simulink model "rigidBodyControl"  (R2016b)
settings: Solver=VariableStepAuto  StartTime=0.0  StopTime=0.4  FixedStep=2e-4  RelTol=1e-3
values from neighbouring files (symbols this model uses):
  denominator = denominator{1}    [mainFeedbackTuning.m]    (also in rigidBodyInit.m)
  denQ = [1 2*wq*0.707 wq*wq]    [rigidBodyInit.m]
  fs = 10000    [mainFeedbackTuning.m]    (also in rigidBodyInit.m = 5000)
  numerator = numerator{1}    [mainFeedbackTuning.m]    (also in rigidBodyInit.m)
  numQ = wq*wq    (= 1421223033.76)    [rigidBodyInit.m]
  Ts = 1/fs    (= 0.0001)    [mainFeedbackTuning.m]    (also in rigidBodyInit.m = 0.0002)
undefined symbols (not defined in the file): m0
libraries: simulink x3, model_controller x1
settings Model: Creator=Dai Luyao  LastModifiedBy=Dai Luyao

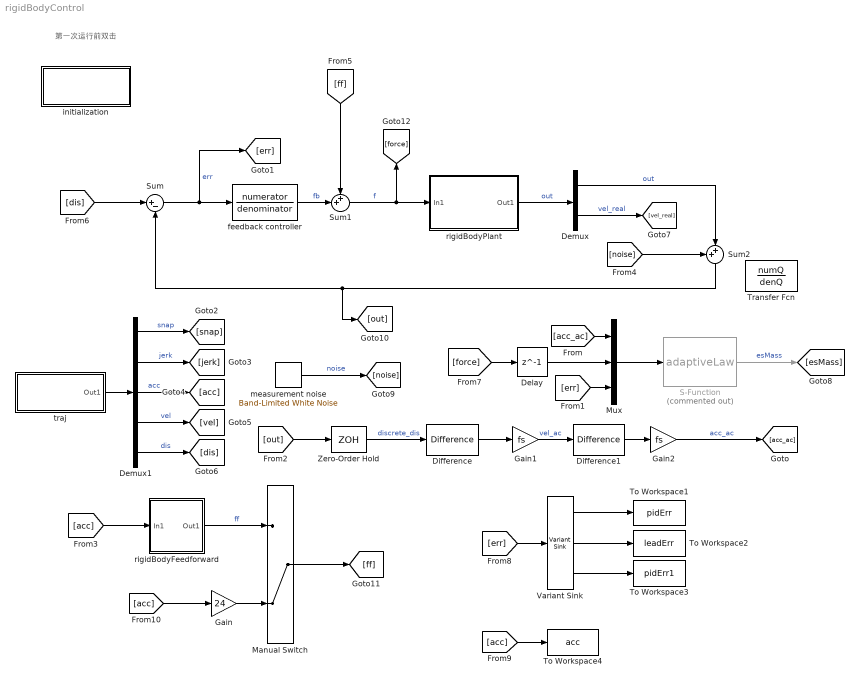
== system rigidBodyControl ==
  note: 第一次运行前双击
  Delay : Delay  DelayLength=1
  Demux : Demux  Outputs=2
  Demux1 : Demux  Outputs=5
  Difference : simulink/Discrete/Difference  ICPrevInput=0.0  OutMin=[]  OutMax=[]  OutDataType=fixdt(1, 16)  OutScaling=2^-10  DoSatur=off
  Difference1 : simulink/Discrete/Difference  ICPrevInput=0.0  OutMin=[]  OutMax=[]  OutDataType=fixdt(1, 16)  OutScaling=2^-10  DoSatur=off
  Gain : Gain  Gain=24
  Gain1 : Gain  Gain=fs
  Gain2 : Gain  Gain=fs
  Manual Switch : ManualSwitch  CurrentSetting=0
  Mux : Mux  Inputs=3
  S-Function : S-Function  Commented=on  FunctionName=adaptiveLaw  Parameters=0.995  SFunctionDeploymentMode=off  EnableBusSupport=off
  Sum : Sum  Inputs=|+-
  Sum1 : Sum  Inputs=++|
  Sum2 : Sum  Inputs=++|
  To Workspace1 : ToWorkspace  VariableName=pidErr  SaveFormat=Structure With Time  SampleTime=-1
  To Workspace2 : ToWorkspace  VariableName=leadErr  SaveFormat=Structure With Time  SampleTime=-1
  To Workspace3 : ToWorkspace  VariableName=pidErr1  SaveFormat=Structure With Time  SampleTime=-1
  To Workspace4 : ToWorkspace  VariableName=acc  SaveFormat=Structure With Time  SampleTime=-1
  Transfer Fcn : TransferFcn  Numerator=numQ  Denominator=denQ
  Variant Sink : VariantSink
  Zero-Order Hold : ZeroOrderHold  SampleTime=Ts
  feedback controller : TransferFcn  Numerator=numerator  Denominator=denominator
  initialization : Subsystem
      settings: OpenFcn=rigidBodyInit;  MoveFcn=edit rigidBodyInit;
  measurement noise : simulink/Sources/Band-Limited White Noise  Cov=noisePower  Ts=Ts  seed=[23341]
  rigidBodyFeedforward : Subsystem
  rigidBodyPlant : Subsystem  mask{m=m0}
      mask prompts: m "mass/kg"
  traj : Subsystem  BlockChoice=4th order traj
      link override 3rd order traj: j=800  v=0.25  x=0.06  a=10
      settings: AttributesFormatString=%<BlockChoice>  TemplateBlock=model_controller/Profile Generators/traj  MemberBlocks=2th order traj,3rd order traj,4th order traj,step
  wires:
  Sum/1 -> feedback controller/1, [err]  "err"
  feedback controller/1 -> Sum1/2  "fb"
  Sum1/1 -> rigidBodyPlant/1(In1), [force]  "f"
  Difference1/1 -> Gain2/1
  Difference/1 -> Gain1/1
  Gain1/1 -> Difference1/1  "vel_ac"
  rigidBodyPlant/1(Out1) -> Demux/1  "out"
  Mux/1 -> S-Function/1
  S-Function/1 -> [esMass]  "esMass"
  [acc_ac] -> Mux/1
  Zero-Order Hold/1 -> Difference/1  "discrete_dis"
  [err] -> Mux/3
  Delay/1 -> Mux/2
  [dis] -> Sum/1
  [acc] -> rigidBodyFeedforward/1(In1)
  Demux/2 -> [vel_real]  "vel_real"
  measurement noise/1 -> [noise]  "noise"
  Demux/1 -> Sum2/2  "out"
  [noise] -> Sum2/1
  Sum2/1 -> [out], Sum/2
  Demux1/1 -> [snap]  "snap"
  Demux1/2 -> [jerk]  "jerk"
  Demux1/3 -> [acc]  "acc"
  Demux1/4 -> [vel]  "vel"
  Demux1/5 -> [dis]  "dis"
  traj/1(Out1) -> Demux1/1
  [out] -> Zero-Order Hold/1
  rigidBodyFeedforward/1(Out1) -> Manual Switch/1  "ff"
  [force] -> Delay/1
  [err] -> Variant Sink/1
  Variant Sink/1 -> To Workspace1/1
  Variant Sink/2 -> To Workspace2/1
  Variant Sink/3 -> To Workspace3/1
  [acc] -> To Workspace4/1
  Manual Switch/1 -> [ff]
  [acc] -> Gain/1
  Gain/1 -> Manual Switch/2
  Gain2/1 -> [acc_ac]  "acc_ac"
  [ff] -> Sum1/1

== system rigidBodyControl/initialization ==

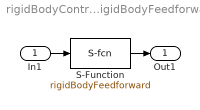
== system rigidBodyControl/rigidBodyFeedforward ==
  In1 : Inport
  S-Function : S-Function  FunctionName=rigidBodyFeedforward  SFunctionDeploymentMode=off  EnableBusSupport=off
  Out1 : Outport
  wires:
  In1/1 -> S-Function/1
  S-Function/1 -> Out1/1

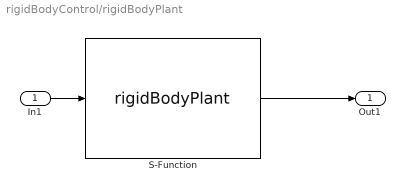
== system rigidBodyControl/rigidBodyPlant ==
  In1 : Inport
  S-Function : S-Function  FunctionName=rigidBodyPlant  Parameters=m  SFunctionDeploymentMode=off  EnableBusSupport=off
  Out1 : Outport
  wires:
  In1/1 -> S-Function/1
  S-Function/1 -> Out1/1

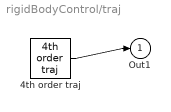
== system rigidBodyControl/traj ==
  4th order traj : model_controller/Profile Generators/4th order traj  t0=0  x=0.06  v=0.25  a=10  j=800  d=64000  Ts=0
  Out1 : Outport
  wires:
  4th order traj/1 -> Out1/1
